simulink library "I2t"  (R2016b)
settings: Solver=VariableStepAuto  StartTime=0.0  StopTime=10.0  RelTol=1e-3
settings Model: Creator=Nathan  LastModifiedBy=march

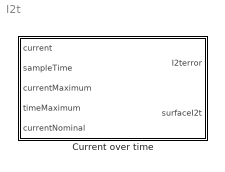
== system I2t ==
  Current over time : Subsystem  ClipboardFcn=I2tLib

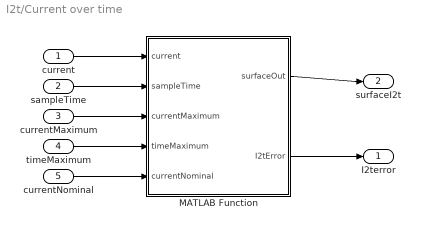
== system I2t/Current over time ==
  current : Inport
  sampleTime : Inport  Port=2
  currentMaximum : Inport  Port=3
  timeMaximum : Inport  Port=4
  currentNominal : Inport  Port=5
  MATLAB Function : MATLAB Function  TreatAsAtomicUnit=on
  I2terror : Outport  BusOutputAsStruct=on
  surfaceI2t : Outport  Port=2
  wires:
  MATLAB Function/2(I2tError) -> I2terror/1
  current/1 -> MATLAB Function/1(current)
  sampleTime/1 -> MATLAB Function/2(sampleTime)
  MATLAB Function/1(surfaceOut) -> surfaceI2t/1
  currentMaximum/1 -> MATLAB Function/3(currentMaximum)
  currentNominal/1 -> MATLAB Function/5(currentNominal)
  timeMaximum/1 -> MATLAB Function/4(timeMaximum)

== matlab function I2t/Current over time/MATLAB Function ==
  data: surfaceOut output; current input; I2tError output; sampleTime input; currentMaximum input; timeMaximum input; currentNominal input
function [surfaceOut, I2tError] = fcn(current,sampleTime, currentMaximum, timeMaximum, currentNominal  )

%% Initialize parameter
persistent surface
persistent prevError;

% If the surface is still empty set it to 0
if isempty(surface) 
    surface = 0;
    prevError = 0;
end

% Time step from the SLRT model, should not be defined here
timeStep = sampleTime; %[s]

% The maximum I2t surafeca can be found
surfaceMaximum = timeMaximum * (currentMaximum^2 - currentNominal^2); %[I^2*t]

% The I2t value is intergrated
surface = surface + timeStep * (current^2-currentNominal^2);

% Determine whether we are in a danger zone or not
if prevError == 0
    if surface > surfaceMaximum
        I2tError = 1;
    else
        I2tError = 0;
    end
else
    if surface > 0.5 * surfaceMaximum
        I2tError = 1;
    else
        I2tError = 0;
    end
end

% surface should never be lower than 0
if surface < 0
    surface = 0;
end

surfaceOut = surface;
prevError = I2tError;
